simulink model "Final_V620140905h5b_fuben1"  (Simulink 7.9)
settings: Solver=FixedStepDiscrete  StartTime=0.0  StopTime=1  FixedStep=Auto  RelTol=1e-3
undefined symbols (not defined in the file or in its folder): Down, Up
libraries: tiiqmathlib x157, idelinklib_common x83, c2833xlib x37, simulink x12, c28xdmclib x12, c280xlib x7, simulink_extras x4, commutil2 x2, idelinklib_tgtpref x1, idelinklib_ticcs x1
(part 7 of 7)

== stateflow chart Function-Call Subsystem1/Control Logic2 ==
  state state0
    during: Out=0;
  state state3
    during: Out=1; F3=1; F1=0; F2=0; F4=0; F5=0; F6=0;
  state state2
    during: Out=1; F2=1; F1=0; F3=0; F4=0; F5=0; F6=0;
  state state1
    during: Out=1;F1=1; F2=0; F3=0; F4=0; F5=0; F6=0;
  state state7
    entry: F1=0; F2=0; F3=0; F4=0; F5=0; F6=0;
  state state4
    during: Out=1; F4=1; F1=0; F2=0; F3=0; F5=0; F6=0;
  state state5
    during: Out=1; F5=1; F1=0; F2=0; F3=0; F4=0; F6=0;
  state state6
    during: Out=1; F6=1; F1=0; F2=0; F3=0; F4=0; F5=0;
  (default) -> state7
  state0 -> state2 [order 1] : [state==0&&Vg1==1&&Vg2==0&&F2==0]
  state2 -> state0 : [K>=0.95]
  state0 -> state3 [order 2] : [state==0&&Vg1==0&&Vg2==1&&F3==0]
  state3 -> state0 : [K>=0.95]
  state1 -> state0 : [K>=0.95]
  state0 -> state1 [order 3] : [state==0&&Vg1==0&&Vg2==0&&F1==0]
  state7 -> state0
  state0 -> state3 [order 4] : [state==0&&Vg1==1&&Vg2==1&&F3==0]
  state0 -> state4 [order 5] : [state==5&&F4==0]
  state0 -> state5 [order 6] : [state==10&&F5==0]
  state0 -> state6 [order 7] : [state==11&&F6==0]
  state4 -> state0 : [K>=0.95]
  state5 -> state0 : [K>=0.95]
  state6 -> state0 : [K>=0.95]
  data: Vg1 input uint16; Vg2 input uint16; Out output fixdt(1,32,16); F1 local uint16; F2 local uint16; F3 local uint16; state input uint16; K input fixdt(1,32,16); F4 local uint16; F5 local uint16; F6 local uint16
